simulink library "dspelem2"  (Simulink 3.00)
undefined symbols (not defined in the file or in its folder): magnitude
libraries: dspmtrx2 x1
settings Model: Creator=don  LastModifiedBy=thartley

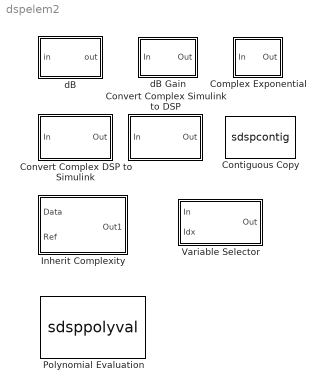
== system dspelem2 ==
  Complex Exponential : Subsystem
      mask Type: Complex Exponential
      mask Description:
      | Compute the complex exponential function of real inputs via
      | Euler's formula, y = cos(x)+jsin(x).
      mask Help: web(dspbhelp);
      mask Display: text(0.2, 0.55,'exp(jx)');
  Contiguous Copy : S-Function  FunctionName=sdspcontig  PortCounts=[]  SFunctionModules=''
      mask Type: Contiguous Copy
      mask Description: Create a contiguous copy of input data.  For use with blocks that only accept contiguous data during simulation or code generation.
      mask Help: web(dspbhelp);
      mask Display: disp('Contiguous\nCopy');
  Convert Complex DSP to Simulink : Subsystem  mask(Convert Complex DSP To Simulink){}
      mask help: Convert old DSP Blockset (prior to V3.0) complex data format to new Simulink complex data type.
      mask init:
      | [x,y]=cplxico2([],1);
      mask Help: web(dspbhelp);
      mask Display:
      | plot(x,y)
      | text(90,50,'Convert\nComplex','horiz','right');
  "Convert Complex Simulink to DSP " : Subsystem  mask(Convert Complex Simulink to DSP){}
      mask help: Convert new Simulink complex data type to old DSP Blockset (prior to V3.0) complex data format.
      mask init:
      | [x,y]=cplxico2(1,[]);
      mask Help: web(dspbhelp);
      mask Display:
      | plot(x,y);
      | text(10,50,'Convert\nComplex','horiz','left');
  Inherit Complexity : Subsystem
      mask Type: Inherit Complexity
      mask Description: Copy data from the Data input with the complexity of the reference signal. If the data is real and the reference is complex, an all zero imaginary part is created. If the data is complex and the reference is real, the imaginary part of the input is removed.
      mask Help: web(dspbhelp);
      mask Display: text(.9,0.5,'Inherit\nComplexity','horiz','right');
  Polynomial Evaluation : S-Function  FunctionName=sdsppolyval  Parameters=constCoeffs,useConstCoeffs  PortCounts=[]  SFunctionModules=''  mask(Polynomial Evaluation){useConstCoeffs=off, constCoeffs=[5 4 3 2 1]}
      mask prompts: useConstCoeffs "Use constant coefficients"; constCoeffs "Constant coefficients:"
      mask help:
      | Apply specified polynomial function to input.
      |
      | Example: [1 3 5] represents u^2 + 3u + 5.
      mask init:
      | [p,xy] = dspblkpolyval('icon');
      mask Help: web(dspbhelp);
      mask CallbackString: dspblkpolyval|
      mask Display:
      | port_label(p.in1,   p.i1,  p.i1s);
      | port_label(p.in2,   p.i2,  p.i2s);
      | port_label(p.out, p.o1, p.o1s);
      | disp(xy.blklabel)
  Variable Selector : Subsystem  mask(Variable Selector){IdxMode=Variable, Elements=[1 3], errmode=Clip and Warn}
      mask prompts: IdxMode "Selector mode:"; errmode "Invalid index:"
      mask help:
      | Select or re-order the specified elements of the input vector.
      | y=u[Elements].
      | Elements may be constant (fixed), or may change throughout the simulation (variable).  Elements are 1-based indices, and do not need to be unique.
      mask init:
      | dspblkvarsel('init');
      mask Help: web(dspbhelp);
      mask StyleString: popup(Fixed|Variable),edit,popup(Clip Index|Clip and Warn|Generate Error)
      mask CallbackString: dspblkvarsel;||
      mask Display: disp('Selector')
  dB : Subsystem  mask(dB){dBtype=dB, intype=Amplitude, R=1, fuzz=on}
      mask prompts: dBtype "Convert to:"; intype "Input signal:"; R "Load resistance (ohms):"; fuzz "Add  eps to input to protect against  "log(0) = -inf""
      mask help: Convert input of Watts or Volts to decibels. Voltage inputs are first converted to power relative to the specified load resistance, where P = (V^2)/R. When converting to dBm, the power is scaled to units of mWatts.
      mask init:
      | str = dspblkdb('init');
      | dspblkdb('checkparam');
      | dspblkdb('update');
      mask Help: web(dspbhelp);
      mask StyleString: popup(dB|dBm),popup(Power|Amplitude),edit,checkbox
      mask CallbackString: dspblkdb;|dspblkdb;||
      mask Display: disp(str)
  dB Gain : Subsystem  mask(dB Gain){dB=-40, intype=Amplitude}
      mask prompts: dB "Gain, dB:"; intype "Input signal:"
      mask help: Apply a gain specified in dB.
      mask init:
      | if isempty(dB),
      |   dB = 0; g = 0;
      |    s = [&1 ' dB'];
      | else
      |   g=10.^(dB/(10*intype));
      |   s = sprintf('%g dB\n(%g)',dB,g);
      | end
      mask Help: web(dspbhelp);
      mask StyleString: edit,popup(Power|Amplitude)
      mask Display: fprintf(s)

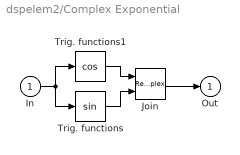
== system dspelem2/Complex Exponential ==
  In : Inport  Port=1  PortWidth=-1  SampleTime=-1  DataType=auto
      settings: SignalType=auto
  Join : RealImagToComplex  Input=RealAndImag  ConstantPart=0
  Trig. functions : Trigonometry  Operator=sin  OutputSignalType=auto
  Trig. functions1 : Trigonometry  Operator=cos  OutputSignalType=auto
  Out : Outport  Port=1  InitialOutput=0
  wires:
  Trig. functions/1 -> Join/2
  Trig. functions1/1 -> Join/1
  Join/1 -> Out/1
  In/1 -> Trig. functions/1, Trig. functions1/1

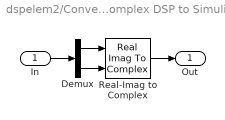
== system dspelem2/Convert Complex DSP to Simulink ==
  In : Inport  Port=1  PortWidth=-1  SampleTime=-1  DataType=auto
      settings: SignalType=auto
  Demux : Demux  Outputs=2
  Real-Imag to Complex : RealImagToComplex  Input=RealAndImag  ConstantPart=0
  Out : Outport  Port=1
  wires:
  In/1 -> Demux/1
  Real-Imag to Complex/1 -> Out/1
  Demux/2 -> Real-Imag to Complex/2
  Demux/1 -> Real-Imag to Complex/1

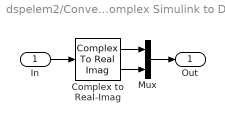
== system dspelem2/Convert Complex Simulink to DSP  ==
  In : Inport  Port=1  PortWidth=-1  SampleTime=-1  DataType=auto
      settings: SignalType=auto
  Complex to Real-Imag : ComplexToRealImag  Output=RealAndImag
  Mux : Mux  Inputs=2
  Out : Outport  Port=1
  wires:
  Mux/1 -> Out/1
  In/1 -> Complex to Real-Imag/1
  Complex to Real-Imag/2 -> Mux/2
  Complex to Real-Imag/1 -> Mux/1

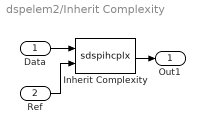
== system dspelem2/Inherit Complexity ==
  Data : Inport  Port=1  PortWidth=-1  SampleTime=-1  DataType=auto
      settings: SignalType=auto
  Ref : Inport  Port=2  PortWidth=-1  SampleTime=-1  DataType=auto
      settings: SignalType=auto
  Inherit Complexity : S-Function  FunctionName=sdspihcplx  PortCounts=[]  SFunctionModules=''
  Out1 : Outport  Port=1
  wires:
  Inherit Complexity/1 -> Out1/1
  Data/1 -> Inherit Complexity/1
  Ref/1 -> Inherit Complexity/2

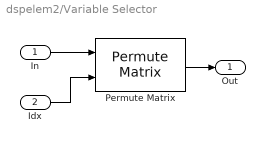
== system dspelem2/Variable Selector ==
  In : Inport  Port=1  PortWidth=-1  SampleTime=-1  DataType=auto
      settings: SignalType=auto
  Idx : Inport  Port=2  PortWidth=-1  SampleTime=-1  DataType=auto
      settings: SignalType=auto
  Permute Matrix : dspmtrx2/Permute Matrix  mode=Rows  errmode=Clip and Warn  cols=1
  Out : Outport  Port=1
  wires:
  In/1 -> Permute Matrix/1
  Permute Matrix/1 -> Out/1
  Idx/1 -> Permute Matrix/2

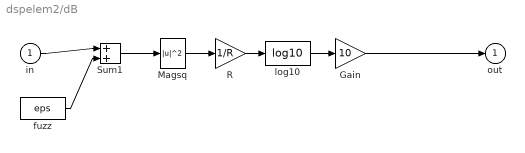
== system dspelem2/dB ==
  in : Inport  Port=1  PortWidth=-1  SampleTime=-1  DataType=auto
      settings: SignalType=auto
  Gain : Gain  Gain=10  SaturateOnIntegerOverflow=on
  Magsq : Math  Operator=magnitude^2  OutputSignalType=auto
  R : Gain  Gain=1/R  SaturateOnIntegerOverflow=on
  Sum1 : Sum  Inputs=++  SaturateOnIntegerOverflow=on
  fuzz : Constant  Value=eps
  log10 : Math  Operator=log10  OutputSignalType=auto
  out : Outport  Port=1  InitialOutput=0
  wires:
  log10/1 -> Gain/1
  Magsq/1 -> R/1
  R/1 -> log10/1
  in/1 -> Sum1/1
  Sum1/1 -> Magsq/1
  fuzz/1 -> Sum1/2
  Gain/1 -> out/1

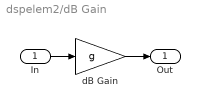
== system dspelem2/dB Gain ==
  In : Inport  Port=1  PortWidth=-1  SampleTime=-1  DataType=auto
      settings: SignalType=auto
  dB Gain : Gain  Gain=g  SaturateOnIntegerOverflow=on
  Out : Outport  Port=1  InitialOutput=0
  wires:
  dB Gain/1 -> Out/1
  In/1 -> dB Gain/1
